simulink model "Model24"  (R2020a)
settings: Solver=VariableStepAuto  StartTime=0.0  StopTime=2  RelTol=1e-3
values from neighbouring files (symbols this model uses):
  b = 3.5077E-6    [DD24.sldd]
  J = 3.2284E-6    [DD24.sldd]
  K = 0.0274    [DD24.sldd]
  L = 2.75E-6    [DD24.sldd]
  R = 4.0    [DD24.sldd]
settings Model: DataDictionary=DD24.sldd  Creator=HP  LastModifiedBy=HP

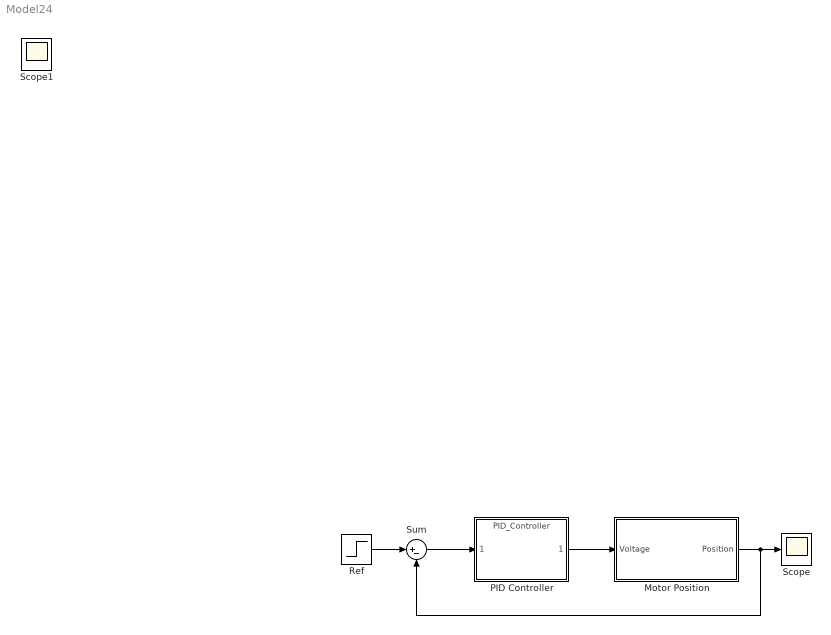
== system Model24 ==
  Motor Position : Subsystem
  PID Controller : ModelReference  ModelNameDialog=PID_Controller  ModelReferenceVersion=1.5
  Ref : Step  SampleTime=0
  Scope : Scope
  Sum : Sum  Inputs=|+-
  Scope1 : Scope
  wires:
  Motor Position/1(Position) -> Sum/2, Scope/1
  Ref/1 -> Sum/1
  PID Controller/1 -> Motor Position/1(Voltage)
  Sum/1 -> PID Controller/1

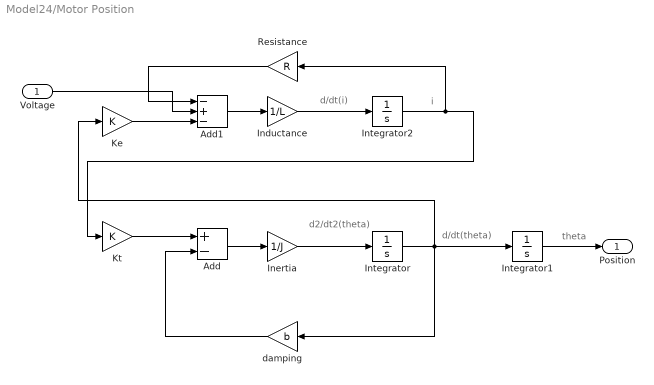
== system Model24/Motor Position ==
  note: i
  note: d2/dt2(theta)
  note: d/dt(theta)
  note: d/dt(i)
  note: theta
  Voltage : Inport
  Add : Sum  Inputs=+-
  Add1 : Sum  Inputs=-+-
  Inductance : Gain  Gain=1/L
  Inertia : Gain  Gain=1/J
  Integrator : Integrator
  Integrator1 : Integrator
  Integrator2 : Integrator
  Ke : Gain  Gain=K
  Kt : Gain  Gain=K
  Resistance : Gain  Gain=R
  damping : Gain  Gain=b
  Position : Outport
  wires:
  Inertia/1 -> Integrator/1
  Kt/1 -> Add/1
  Add1/1 -> Inductance/1
  damping/1 -> Add/2
  Integrator1/1 -> Position/1
  Add/1 -> Inertia/1
  Integrator/1 -> damping/1, Integrator1/1, Ke/1
  Voltage/1 -> Add1/2
  Resistance/1 -> Add1/1
  Ke/1 -> Add1/3
  Integrator2/1 -> Resistance/1, Kt/1
  Inductance/1 -> Integrator2/1
